simulink model "Erdorbits"  (R2015a)
settings: Solver=ode45  StartTime=0.0  StopTime=5780  RelTol=1e-3
settings Model: Creator=leon  LastModifiedBy=leon

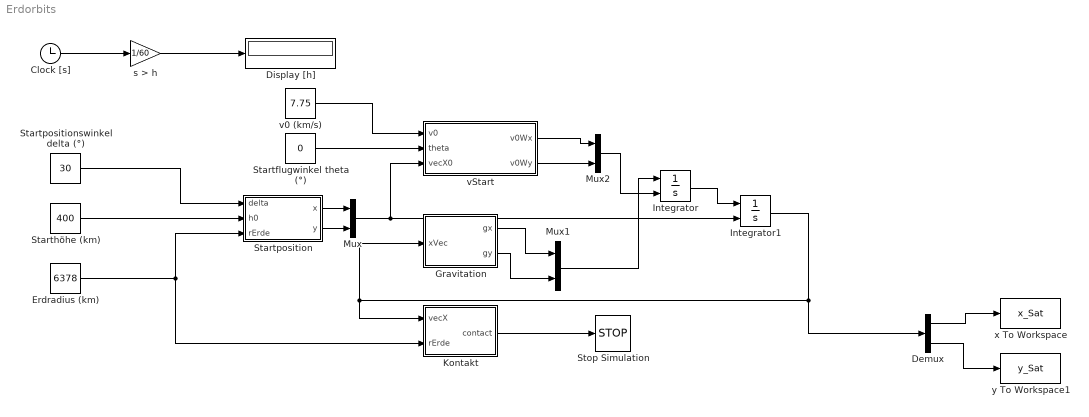
== system Erdorbits ==
  Clock [s] : Clock
  Demux : Demux  Outputs=2
  Display [h] : Display
  "Erdradius (km) " : Constant  Value=6378
  Gravitation : MATLAB Function  TreatAsAtomicUnit=on
  Integrator : Integrator  InitialConditionSource=external
  Integrator1 : Integrator  InitialConditionSource=external
  Kontakt : MATLAB Function  TreatAsAtomicUnit=on
  Mux : Mux  Inputs=2
  Mux1 : Mux  Inputs=2
  Mux2 : Mux  Inputs=2
  Startflugwinkel theta (°) : Constant  Value=0
  Starthöhe (km) : Constant  Value=400
  Startposition : MATLAB Function  TreatAsAtomicUnit=on
  "Startpositionswinkel delta (°) " : Constant  Value=30
  Stop Simulation : Stop
  s > h : Gain  Gain=1/60
  v0 (km/s) : Constant  Value=7.75
  vStart : MATLAB Function  TreatAsAtomicUnit=on
  x To Workspace : ToWorkspace  VariableName=x_Sat  SampleTime=-1
  y To Workspace1 : ToWorkspace  VariableName=y_Sat  SampleTime=-1
  wires:
  Startposition/1(x) -> Mux/1
  "Startpositionswinkel delta (°) "/1 -> Startposition/1(delta)
  Starthöhe (km)/1 -> Startposition/2(h0)
  "Erdradius (km) "/1 -> Kontakt/2(rErde), Startposition/3(rErde)
  Startflugwinkel theta (°)/1 -> vStart/2(theta)
  v0 (km/s)/1 -> vStart/1(v0)
  Clock [s]/1 -> s > h/1
  s > h/1 -> Display [h]/1
  Kontakt/1(contact) -> Stop Simulation/1
  Mux/1 -> vStart/3(vecX0), Integrator1/2
  Startposition/2(y) -> Mux/2
  Demux/1 -> x To Workspace/1
  Demux/2 -> y To Workspace1/1
  Integrator1/1 -> Demux/1, Kontakt/1(vecX), Gravitation/1(xVec)
  Gravitation/2(gy) -> Mux1/2
  Gravitation/1(gx) -> Mux1/1
  vStart/2(v0Wy) -> Mux2/2
  vStart/1(v0Wx) -> Mux2/1
  Mux2/1 -> Integrator/2
  Mux1/1 -> Integrator/1
  Integrator/1 -> Integrator1/1

== matlab function Erdorbits/vStart ==
  data: v0 input; v0Wx output; theta input; vecX0 input; v0Wy output
function [v0Wx, v0Wy]= fcn(v0, theta, vecX0)
%Einheitsvektor Tangentialrichtung
n = vecX0/norm(vecX0);  % Eigentlich - Ursprung
%Einheitsvektor Normalenrichtung
t = [n(2); -n(1)];

%- Tangential-und Normalenkomponente der Startgeschwindigkeit (vt , vn) berechnen
rad = theta*pi/180;  %Umrechnung zu Bogenmaß
vt = v0 * 1000 * cos(rad);
vn = v0 * 1000 * sin(rad);
% aus n, t und (v_t, v_n) die Startgeschwindigkeit VecV0Welt zusammenbauen
v0_vec = (vn*n) + (vt*t);  
v0Wx = v0_vec(1,1);
v0Wy =  v0_vec(2,1);

== matlab function Erdorbits/Startposition ==
  data: delta input; x output; h0 input; rErde input; y output
%Geben Sie eine Embedded-Matlab-(EM)-Funktion „Startposition“ an,
%die aus den Parametern (°), der Starthöhe h 0 (km) sowie der Konstante „Erdradius“
%die Startposition ⃗ berechnet ( Anfangswert für die Position).

function [x,y]= fcn(delta, h0, rErde)
diff = (rErde+h0)*1000; %Umwandunlung in Meter
rad = delta*pi/180; %Umwandlung in Radian

y = (diff)*sin(rad) ;
x = sqrt((diff*diff) - (y*y));

== matlab function Erdorbits/Gravitation ==
  data: xVec input; gx output; gy output
function [gx, gy]= fcn(xVec)
  persistent G mErde; 
  G = 66.743*10^-12;       % Gravitationskonstante m^3/(kg*s^2)
  mErde = 5.9736*10^24;    % Erdmasse in kg
  
  esDist = norm(xVec);  % Entfernung Erde (Mitte) -> Satellit
  
  seNormVec = -xVec/norm(xVec); % Normalenvektor Satellit -> Erde
  
  g = G*(mErde/esDist^2)*seNormVec;        % Erdbeschleunigung
 
 gx = g(1,1);
 gy = g(2,1);

== matlab function Erdorbits/Kontakt ==
  data: vecX input; rErde input; contact output
function contact = fcn(vecX, rErde)
r = norm(vecX);
if r <= (rErde*1000)
  contact = 1;
else
  contact = 0;
end
